simulink model "opti_R2019a"  (R2019a)
settings: Solver=VariableStepAuto  StartTime=0.0  StopTime=10.0  RelTol=1e-3
values from neighbouring files (symbols this model uses):
  k1 = K(1)    [ISEUfunc.m]    (also in ISEfunc.m; ITSEfunc.m; costMpfunc.m; costTr1_100Mp0func.m)
  k2 = K(2)    [ISEUfunc.m]    (also in ISEfunc.m; ITSEfunc.m; costMpfunc.m; costTr1_100Mp0func.m)
settings Model: Creator=Mertcan  LastModifiedBy=Mertcan

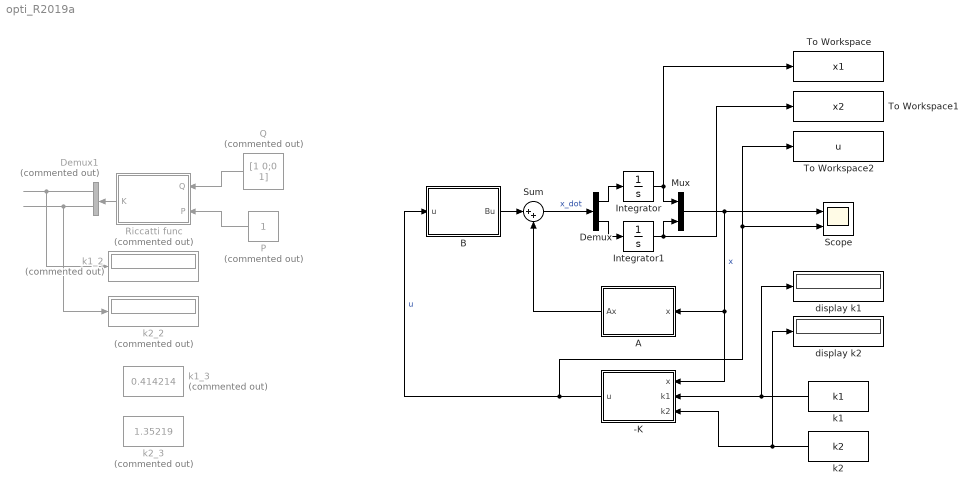
== system opti_R2019a ==
  -K : MATLAB Function  TreatAsAtomicUnit=on
  A : MATLAB Function  TreatAsAtomicUnit=on
  B : MATLAB Function  TreatAsAtomicUnit=on
  Demux : Demux  Outputs=2
  Demux1 : Demux  Commented=on  Outputs=2
  Integrator : Integrator  InitialCondition=1
  Integrator1 : Integrator  InitialCondition=-1
  Mux : Mux  Inputs=2
  P : Constant  Commented=on
  Q : Constant  Commented=on  Value=[1 0;0 1]
  Riccatti func : MATLAB Function  Commented=on  TreatAsAtomicUnit=on
  Scope : Scope  NumInputPorts=2
  Sum : Sum  Inputs=|++
  To Workspace : ToWorkspace  VariableName=x1  SaveFormat=Timeseries  SampleTime=-1
  To Workspace1 : ToWorkspace  VariableName=x2  SaveFormat=Timeseries  SampleTime=-1
  To Workspace2 : ToWorkspace  VariableName=u  SaveFormat=Timeseries  SampleTime=-1
  display k1 : Display
  display k2 : Display
  k1 : Constant  Value=k1
  k1_2 : Display  Commented=on
  k1_3 : Constant  Commented=on  Value=0.414214
  k2 : Constant  Value=k2
  k2_2 : Display  Commented=on
  k2_3 : Constant  Commented=on  Value=1.35219
  wires:
  B/1(Bu) -> Sum/1
  Mux/1 -> Scope/1, A/1(x), -K/1(x)  "x"
  Sum/1 -> Demux/1  "x_dot"
  A/1(Ax) -> Sum/2
  -K/1(u) -> To Workspace2/1, Scope/2, B/1(u)  "u"
  Demux/1 -> Integrator/1
  Demux/2 -> Integrator1/1
  Integrator1/1 -> To Workspace1/1, Mux/2
  Integrator/1 -> Mux/1, To Workspace/1
  Demux1/2 -> k2_2/1
  Demux1/1 -> k1_2/1
  P/1 -> Riccatti func/2(P)
  Q/1 -> Riccatti func/1(Q)
  Riccatti func/1(K) -> Demux1/1
  k1/1 -> -K/2(k1), display k1/1
  k2/1 -> -K/3(k2), display k2/1

== matlab function opti_R2019a/A ==
  data: x input size=2; Ax output size=2
function Ax = A(x)

Ax = [x(2);-x(1)];

== matlab function opti_R2019a/B ==
  data: u input size=1; Bu output size=2
function Bu = B(u)

Bu = [0;u];

== matlab function opti_R2019a/-K ==
  data: x input size=2; u output size=1; k1 input size=1; k2 input size=1
function u = minusK(x,k1,k2)

u = -k1*x(1) - k2*x(2);

== matlab function opti_R2019a/Riccatti func ==
  data: Q input; K output; P input
function K = fcn(Q,P)

A = [0,1;-1,0];
B = [0;1];

R = icare(A,B,Q,P,[],[],[]);

K = R*B;
